simulink model "PID_Controller_MR1"  (R2024b)
settings: Solver=VariableStepAuto  StartTime=0.0  StopTime=10.0  RelTol=1e-3
InitFcn:
  | J =0.01;
  | b = 0.1;
  | K = 0.01;
  | R = 1;
  | kb =0.01;
  | L = 0.5;
  | Kp=550;
  | ki = 500;
  | Ts = 0.01;
  | Kd =0.01;
settings Model: Creator=chall  LastModifiedBy=chall
settings DataIOCC: SaveOutput=off  SaveTime=off

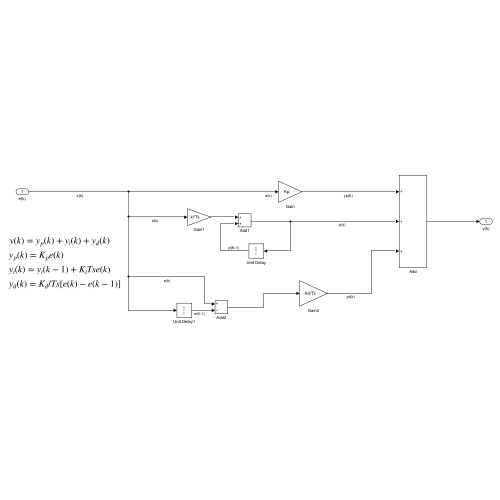
[thumbnail: Simulink's stored preview of the top-level diagram]
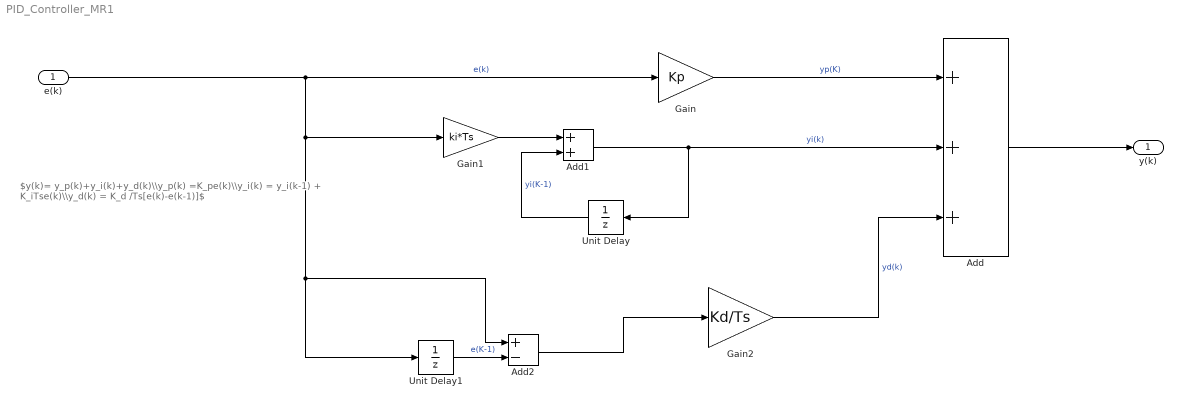
== system PID_Controller_MR1 ==
  note: $y(k)= y_p(k)+y_i(k)+y_d(k)\\y_p(k) =K_pe(k)\\y_i(k) = y_i(k-1) + K_iTse(k)\\y_d(k) = K_d /Ts[e(k)-e(k-1)]$
  e(k) : Inport  OutDataTypeStr=double  PortDimensions=1  SampleTime=0
  Add : Sum  Inputs=+++
  Add1 : Sum
  Add2 : Sum  Inputs=+-
  Gain : Gain  Gain=Kp
  Gain1 : Gain  Gain=ki*Ts
  Gain2 : Gain  Gain=Kd/Ts
  Unit Delay : UnitDelay  SampleTime=-1  HasFrameUpgradeWarning=on
  Unit Delay1 : UnitDelay  SampleTime=-1  HasFrameUpgradeWarning=on
  y(k) : Outport  OutDataTypeStr=double  PortDimensions=1  SampleTime=0
  wires:
  e(k)/1 -> Gain/1, Gain1/1, Unit Delay1/1, Add2/1  "e(k)"
  Gain/1 -> Add/1  "yp(K)"
  Gain1/1 -> Add1/1
  Add1/1 -> Add/2, Unit Delay/1  "yi(k)"
  Unit Delay/1 -> Add1/2  "yi(K-1)"
  Add/1 -> y(k)/1
  Gain2/1 -> Add/3  "yd(k)"
  Unit Delay1/1 -> Add2/2  "e(K-1)"
  Add2/1 -> Gain2/1
